simulink model "ACC_Model"  (Simulink 7.6)
settings: Solver=ode5  StartTime=0.0  StopTime=inf  FixedStep=1/100  RelTol=1e-3
undefined symbols (not defined in the file or in its folder): DiscIntNeverNeededParam
libraries: simulink x21, simulink_extras x6
(part 1 of 4)
settings Model: Creator=Krzysztof  LastModifiedBy=pastora  BufferReuse=off
settings DataIOCC: SaveOutput=off  SaveTime=off
settings OptimizationCC: InlineParams=on  OptimizeBlockIOStorage=off  BufferReuse=off  ExpressionFolding=off  LocalBlockOutputs=off
settings DebuggingCC: SaveWithDisabledLinksMsg=none  SaveWithParameterizedLinksMsg=none  SolverPrmCheckMsg=none  InheritedTsInSrcMsg=none  DiscreteInheritContinuousMsg=none  ParameterPrecisionLossMsg=none
settings ModelReferenceCC: ModelReferenceNumInstancesAllowed=Single
settings SFSimCC: SimParseCustomCode=off

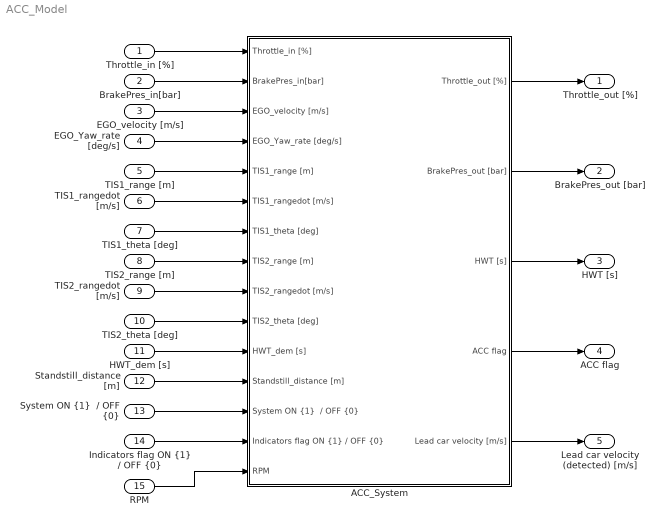
== system ACC_Model ==
  Throttle_in [%] : Inport
  BrakePres_in[bar] : Inport  Port=2
  EGO_velocity [m/s] : Inport  Port=3
  EGO_Yaw_rate [deg/s] : Inport  Port=4
  TIS1_range [m] : Inport  Port=5
  TIS1_rangedot [m/s] : Inport  Port=6
  TIS1_theta [deg] : Inport  Port=7
  TIS2_range [m] : Inport  Port=8
  TIS2_rangedot [m/s] : Inport  Port=9
  TIS2_theta [deg] : Inport  Port=10
  HWT_dem [s] : Inport  Port=11
  Standstill_distance [m] : Inport  Port=12
  "System ON {1}  / OFF {0}" : Inport  Port=13
  "Indicators flag ON {1} / OFF {0}" : Inport  Port=14
  RPM : Inport  Port=15
  ACC_System : Subsystem  mask(ACC System){J_xx=210, Rw=0.34, LaneWidth=3.5, Qfac=40.4695, BrakePressureMax=150, BrakeMax=3.5, MaxSpeed=200, drd=3, LowSpeedActv=40, TISMaxRange=[150 30], TISMaxTheta=[9 80], Tblock=1/100, TISsensor=[1/25 1/25], TISdet=[32 32], DisplaySwitch=on, DisplayFreq=25, RadarSwitch=on, RadarFreq=25}
      mask prompts: J_xx "Principal moment of inertia along longitudal (x) axis Jxx [kg*m^2]"; Rw "Tyre radius Rw [m]"; LaneWidth "Width of the lane [m]"; Qfac "Conversion factor of braking pressure into braking torque Qfac [Nm/bar]"; BrakePressureMax "Maximum brake pressure (that the controller can apply) [bar]"; BrakeMax "Maximum acceleration / deceleration, which can be applied by ACC [m/s^2]"; MaxSpeed "Maximum ACC operating velocity [km/h]"; drd "Cut-Off relatve velocity of EGO and LEAD [km/h]"; LowSpeedActv "LEAD Cut-Off Speed [km/h]"; TISMaxRange "TIS maximum range (TIS1 and TIS2) [m]"; TISMaxTheta "TIS maximum theta angle (TIS1 and TIS2) [deg]"; Tblock "Target update rate of the compilation sheet [s]"; TISsensor "TIS update rate (TIS1 and TIS2) [s]"; TISdet "TIS max. objects to detect (TIS1 and TIS2)"; DisplaySwitch "Show EGO parameters visualization"; DisplayFreq "EGO parameters visualization frequency [Hz]"; RadarSwitch "Show radar visualization"; RadarFreq "Radar frequency [Hz]"
      mask help: PreScan Experiment and Simple Dynamics model parameters
      mask init:
      | Tsensor = max([TISsensor]);
      mask CallbackString:
      | ||||||||||||||en = get_param(gcb,'MaskEnables');
      | switch get_param(gcb, 'DisplaySwitch')
      |     case 'off'
      |         en{16} = 'off';
      |     case 'on'
      |         en{16} = 'on';
      | end
      | set_param(gcb,'MaskEnables',en);||en = get_param(gcb,'MaskEnables');
      | switch get_param(gcb, 'RadarSwitch')
      |     case 'off'
      |         en{18} = 'off';
      |     case 'on'
      |         en{18} = 'on';
      | end
      | set_param(gcb,'MaskEnables',en);|
  Throttle_out [%] : Outport
  BrakePres_out [bar] : Outport  Port=2
  HWT [s] : Outport  Port=3
  ACC flag : Outport  Port=4
  Lead car velocity (detected) [m/s] : Outport  Port=5
  wires:
  "Indicators flag ON {1} / OFF {0}"/1 -> ACC_System/14("Indicators flag ON {1} / OFF {0}")
  ACC_System/1(Throttle_out [%]) -> Throttle_out [%]/1
  ACC_System/2(BrakePres_out [bar]) -> BrakePres_out [bar]/1
  ACC_System/3(HWT [s]) -> HWT [s]/1
  ACC_System/4(ACC flag) -> ACC flag/1
  ACC_System/5(Lead car velocity [m/s]) -> Lead car velocity (detected) [m/s]/1
  EGO_Yaw_rate [deg/s]/1 -> ACC_System/4(EGO_Yaw_rate [deg/s])
  TIS1_range [m]/1 -> ACC_System/5(TIS1_range [m])
  TIS1_rangedot [m/s]/1 -> ACC_System/6(TIS1_rangedot [m/s])
  TIS1_theta [deg]/1 -> ACC_System/7(TIS1_theta [deg])
  TIS2_range [m]/1 -> ACC_System/8(TIS2_range [m])
  TIS2_rangedot [m/s]/1 -> ACC_System/9(TIS2_rangedot [m/s])
  TIS2_theta [deg]/1 -> ACC_System/10(TIS2_theta [deg])
  EGO_velocity [m/s]/1 -> ACC_System/3(EGO_velocity [m/s])
  HWT_dem [s]/1 -> ACC_System/11(HWT_dem [s])
  Standstill_distance [m]/1 -> ACC_System/12(Standstill_distance [m])
  "System ON {1}  / OFF {0}"/1 -> ACC_System/13("System ON {1}  / OFF {0}")
  Throttle_in [%]/1 -> ACC_System/1(Throttle_in [%])
  BrakePres_in[bar]/1 -> ACC_System/2(BrakePres_in[bar])
  RPM/1 -> ACC_System/15(RPM)

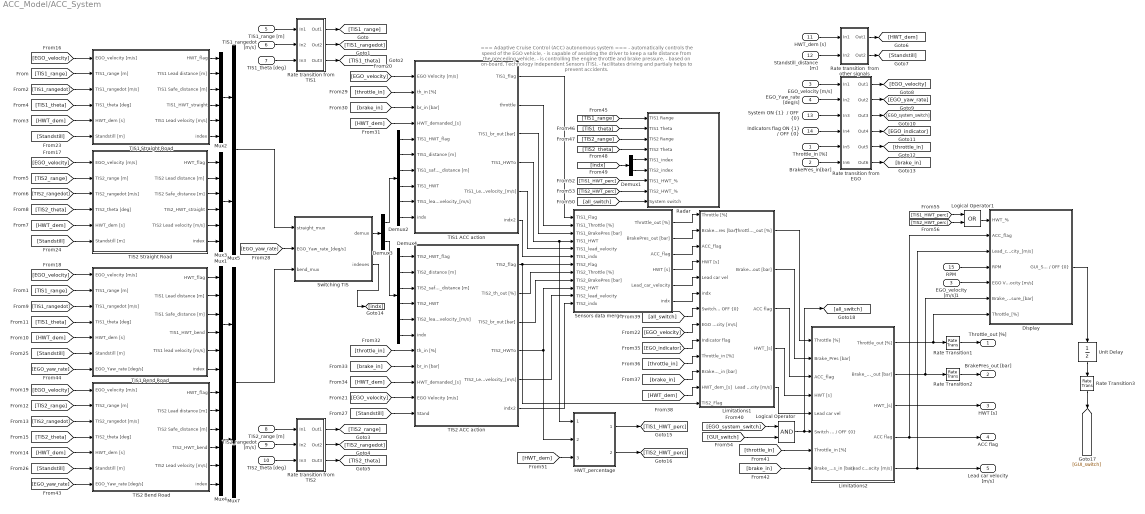
== system ACC_Model/ACC_System ==
  note: === Adaptive Cruise Control (ACC) autonomous system ===
      |
      |  - automatically controls the speed of the EGO vehicle,
      |  - is capable of assisting the driver to keep a safe distance
      |    from the preceding vehicle,
      |  - is controlling the engine throttle and brake pressure,
      |  - based on on-board, Technology Independent Sensors (TIS),
      |  - facilitates driving and partialy helps to prevent accidents.
  Throttle_in [%] : Inport  SampleTime=0
  BrakePres_in[bar] : Inport  Port=2  SampleTime=0
  EGO_velocity [m/s] : Inport  Port=3  SampleTime=Tblock
  EGO_Yaw_rate [deg/s] : Inport  Port=4  SampleTime=Tblock
  TIS1_range [m] : Inport  Port=5  PortDimensions=TISdet(1)  SampleTime=TISsensor(1)
  TIS1_rangedot [m/s] : Inport  Port=6  PortDimensions=TISdet(1)  SampleTime=TISsensor(1)
  TIS1_theta [deg] : Inport  Port=7  PortDimensions=TISdet(1)  SampleTime=TISsensor(1)
  TIS2_range [m] : Inport  Port=8  PortDimensions=TISdet(2)  SampleTime=TISsensor(2)
  TIS2_rangedot [m/s] : Inport  Port=9  PortDimensions=TISdet(2)  SampleTime=TISsensor(2)
  TIS2_theta [deg] : Inport  Port=10  PortDimensions=TISdet(2)  SampleTime=TISsensor(2)
  HWT_dem [s] : Inport  Port=11
  Standstill_distance [m] : Inport  Port=12
  "System ON {1}  / OFF {0}" : Inport  Port=13
  "Indicators flag ON {1} / OFF {0}" : Inport  Port=14
  RPM : Inport  Port=15  SampleTime=0
  Demux1 : Demux  Outputs=2
  Demux2 : Demux  Outputs=6
  Demux3 : Demux  Outputs=2
  Demux4 : Demux  Outputs=6
  Display : Subsystem
  EGO_velocity [m/s]1 : InportShadow  Port=3  SampleTime=Tblock
  HWT_percentage : Subsystem
  Limitations1 : Subsystem
  Limitations2 : Subsystem
  Logical Operator : Logic  AllPortsSameDT=off  OutDataTypeStr=boolean
  Logical Operator1 : Logic  Operator=OR  AllPortsSameDT=off  OutDataTypeStr=boolean
  Mux{1..4} (4 alike) : Mux  Inputs=6
  Mux5 : Mux  Inputs=2
  Mux7 : Mux  Inputs=2
  Radar : Subsystem
  Rate Transition1 : RateTransition  Integrity=off  OutPortSampleTime=0
  Rate Transition2 : RateTransition  Integrity=off  OutPortSampleTime=0
  Rate Transition3 : RateTransition  Integrity=off  OutPortSampleTime=Tsensor
  Rate transition  from other signals : Subsystem
  Rate transition from EGO : Subsystem
  Rate transition from TIS1 : Subsystem
  Rate transition from TIS2 : Subsystem
  Sensors data merge : Subsystem
  Switching TIS : Subsystem
  TIS1 ACC action : Subsystem
  TIS1 Bend Road : Subsystem
  TIS1 Straight Road : Subsystem
  TIS2 ACC action : Subsystem
  TIS2 Bend Road : Subsystem
  TIS2 Straight Road : Subsystem
  Unit Delay : UnitDelay  X0=1  SampleTime=-1
  Throttle_out [%] : Outport
  BrakePres_out [bar] : Outport  Port=2
  HWT [s] : Outport  Port=3
  ACC flag : Outport  Port=4
  Lead car velocity [m/s] : Outport  Port=5
  wires:
  Sensors data merge/1(Throttle_out [%]) -> Limitations1/1(Throttle [%])
  Sensors data merge/2(BrakePres_out [bar]) -> Limitations1/2(Brake_Pres [bar])
  TIS1 ACC action/1(TIS1_flag) -> Sensors data merge/1(TIS1_Flag)
  TIS1 ACC action/2(throttle) -> Sensors data merge/2(TIS1_Throttle [%])
  TIS1 ACC action/3(TIS1_br_out [bar]) -> Sensors data merge/3(TIS1_BrakePres [bar])
  TIS1 ACC action/4(TIS1_HWTo) -> Sensors data merge/4(TIS1_HWT), HWT_percentage/1(TIS1_HWT)
  Sensors data merge/3(ACC_flag) -> Limitations1/3(ACC_flag)
  Sensors data merge/4(HWT [s]) -> Limitations1/4(HWT [s])
  Sensors data merge/5(Lead_car_velocity) -> Limitations1/5(Lead car vel)
  TIS1 ACC action/5(TIS1_Lead_velocity_[m/s]) -> Sensors data merge/5(TIS1_lead_velocity)
  TIS2 ACC action/1(TIS2_flag) -> Sensors data merge/7(TIS2_Flag), Limitations1/13(TIS2_Flag)
  TIS2 ACC action/2(TIS2_th_out [%]) -> Sensors data merge/8(TIS2_Throttle [%])
  TIS2 ACC action/3(TIS2_br_out [bar]) -> Sensors data merge/9(TIS2_BrakePres [bar])
  TIS2 ACC action/4(TIS2_HWTo) -> Sensors data merge/10(TIS2_HWT), HWT_percentage/2(TIS2_HWT)
  TIS2 ACC action/5(TIS2_Lead_velocity_[m/s]) -> Sensors data merge/11(TIS2_lead_velocity)
  TIS1 Straight Road/1(HWT_flag) -> Mux2/1
  TIS1 Straight Road/2(TIS1 Lead distance [m]) -> Mux2/2
  TIS1 Straight Road/3(TIS1 Safe_distance [m]) -> Mux2/3
  TIS1 Straight Road/4(TIS1_HWT_straight) -> Mux2/4
  TIS1 Straight Road/5(TIS1 Lead velocity [m/s]) -> Mux2/5
  TIS1 Straight Road/6(index) -> Mux2/6
  TIS1 ACC action/6(indx2) -> Sensors data merge/6(TIS1_indx)
  TIS2 ACC action/6(indx2) -> Sensors data merge/12(TIS2_indx)
  Sensors data merge/6(indx) -> Limitations1/6(indx)
  Limitations1/1(Throttle_out [%]) -> Limitations2/1(Throttle [%])
  Limitations1/2(Brake_Pres_out [bar]) -> Limitations2/2(Brake_Pres [bar])
  Limitations1/4(HWT_[s]) -> Limitations2/4(HWT [s])
  Limitations1/3(ACC flag) -> Limitations2/3(ACC_flag)
  Limitations1/5(Lead car velocity [m/s]) -> Limitations2/5(Lead car vel)
  TIS1_range [m]/1 -> Rate transition from TIS1/1(In1)
  TIS1_rangedot [m/s]/1 -> Rate transition from TIS1/2(In2)
  TIS1_theta [deg]/1 -> Rate transition from TIS1/3(In3)
  TIS2_range [m]/1 -> Rate transition from TIS2/1(In1)
  TIS2_rangedot [m/s]/1 -> Rate transition from TIS2/2(In2)
  TIS2_theta [deg]/1 -> Rate transition from TIS2/3(In3)
  Rate transition from TIS1/1(Out1) -> [TIS1_range]
  Rate transition from TIS1/2(Out2) -> [TIS1_rangedot]
  Rate transition from TIS1/3(Out3) -> [TIS1_theta]
  Rate transition from TIS2/1(Out1) -> [TIS2_range]
  Rate transition from TIS2/2(Out2) -> [TIS2_rangedot]
  Rate transition from TIS2/3(Out3) -> [TIS2_theta]
  [TIS1_range] -> TIS1 Straight Road/2(TIS1_range [m])
  [TIS1_rangedot] -> TIS1 Straight Road/3(TIS1_rangedot [m/s])
  [TIS1_theta] -> TIS1 Straight Road/4(TIS1_theta [deg])
  [TIS2_range] -> TIS2 Straight Road/2(TIS2_range [m])
  [TIS2_rangedot] -> TIS2 Straight Road/3(TIS2_rangedot [m/s])
  [TIS2_theta] -> TIS2 Straight Road/4(TIS2_theta [deg])
  [TIS1_range] -> TIS1 Bend Road/2(TIS1_range [m])
  [TIS1_rangedot] -> TIS1 Bend Road/3(TIS1_rangedot [m/s])
  [TIS1_theta] -> TIS1 Bend Road/4(TIS1_theta [deg])
  [TIS2_range] -> TIS2 Bend Road/2(TIS2_range [m])
  [TIS2_rangedot] -> TIS2 Bend Road/3(TIS2_rangedot [m/s])
  [TIS2_theta] -> TIS2 Bend Road/4(TIS2_theta [deg])
  EGO_velocity [m/s]/1 -> Rate transition from EGO/1(In1)
  EGO_Yaw_rate [deg/s]/1 -> Rate transition from EGO/2(In2)
  HWT_dem [s]/1 -> Rate transition  from other signals/1(In1)
  Standstill_distance [m]/1 -> Rate transition  from other signals/2(In2)
  "System ON {1}  / OFF {0}"/1 -> Rate transition from EGO/3(In3)
  Throttle_in [%]/1 -> Rate transition from EGO/5(In5)
  BrakePres_in[bar]/1 -> Rate transition from EGO/6(In6)
  "Indicators flag ON {1} / OFF {0}"/1 -> Rate transition from EGO/4(In4)
  Rate transition  from other signals/1(Out1) -> [HWT_dem]
  Rate transition  from other signals/2(Out2) -> [Standstill]
  [HWT_dem] -> TIS1 Straight Road/5(HWT_dem [s])
  [HWT_dem] -> TIS2 Straight Road/5(HWT_dem [s])
  [HWT_dem] -> TIS1 Bend Road/5(HWT_dem [s])
  [HWT_dem] -> TIS2 Bend Road/5(HWT_dem [s])
  Rate transition from EGO/1(Out1) -> [EGO_velocity]
  Rate transition from EGO/2(Out2) -> [EGO_yaw_rate]
  Rate transition from EGO/3(Out3) -> [EGO_system_switch]
  Rate transition from EGO/4(Out4) -> [EGO_indicator]
  Rate transition from EGO/5(Out5) -> [throttle_in]
  Rate transition from EGO/6(Out6) -> [brake_in]
  [EGO_velocity] -> TIS1 Straight Road/1(EGO_velocity [m/s])
  [EGO_velocity] -> TIS2 Straight Road/1(EGO_velocity [m/s])
  [EGO_velocity] -> TIS1 Bend Road/1(EGO_velocity [m/s])
  [EGO_velocity] -> TIS2 Bend Road/1(EGO_velocity [m/s])
  [EGO_velocity] -> TIS1 ACC action/1(EGO Velocity [m/s])
  [EGO_velocity] -> TIS2 ACC action/10(EGO Velocity [m/s])
  [EGO_velocity] -> Limitations1/8(EGO Velocity [m/s])
  [Standstill] -> TIS1 Straight Road/6(Standstill [m])
  [Standstill] -> TIS2 Straight Road/6(Standstill [m])
  [Standstill] -> TIS1 Bend Road/6(Standstill [m])
  [Standstill] -> TIS2 Bend Road/6(Standstill [m])
  [Standstill] -> TIS2 ACC action/11(Stand)
  [EGO_yaw_rate] -> Switching TIS/2(EGO_Yaw_rate_[deg/s])
  [throttle_in] -> TIS1 ACC action/2(th_in [%])
  [brake_in] -> TIS1 ACC action/3(br_in [bar])
  [HWT_dem] -> TIS1 ACC action/4(HWT_demanded_[s])
  [throttle_in] -> TIS2 ACC action/7(th_in [%])
  [brake_in] -> TIS2 ACC action/8(br_in [bar])
  [HWT_dem] -> TIS2 ACC action/9(HWT_demanded_[s])
  [EGO_indicator] -> Limitations1/9(Indicator flag)
  [throttle_in] -> Limitations1/10(Throttle_in [%])
  [brake_in] -> Limitations1/11(Brake_Pres_in [bar])
  [HWT_dem] -> Limitations1/12(HWT_dem_[s])
  [all_switch] -> Limitations1/7("Switch ON {1} / OFF {0}")
  [throttle_in] -> Limitations2/7(Throttle_in [%])
  [brake_in] -> Limitations2/8(Brake_Pres_in [bar])
  [EGO_yaw_rate] -> TIS2 Bend Road/7(EGO_Yaw_rate [deg/s])
  [EGO_yaw_rate] -> TIS1 Bend Road/7(EGO_Yaw_rate [deg/s])
  Limitations2/1(Throttle_out [%]) -> Rate Transition1/1, Display/7(Throttle_[%])
  Limitations2/2(Brake_Pres_out [bar]) -> Rate Transition2/1, Display/6(Brake_Pressure_[bar])
  Rate Transition1/1 -> Throttle_out [%]/1
  Rate Transition2/1 -> BrakePres_out [bar]/1
  Limitations2/3(HWT_[s]) -> HWT [s]/1
  Limitations2/4(ACC flag) -> ACC flag/1, Display/2(ACC_flag)
  Limitations2/5(Lead car velocity [m/s]) -> Lead car velocity [m/s]/1, Display/3(Lead_car_velocity_[m/s])
  [TIS1_range] -> Radar/1(TIS1 Range)
  [TIS1_theta] -> Radar/2(TIS1 Theta)
  [TIS2_range] -> Radar/3(TIS2 Range)
  [TIS2_theta] -> Radar/4(TIS2 Theta)
  Mux2/1 -> Mux5/1
  TIS2 Straight Road/1(HWT_flag) -> Mux3/1
  TIS2 Straight Road/2(TIS2 Lead distance [m]) -> Mux3/2
  TIS2 Straight Road/3(TIS2 Safe_distance [m]) -> Mux3/3
  TIS2 Straight Road/4(TIS2_HWT_straight) -> Mux3/4
  TIS2 Straight Road/5(TIS2 Lead velocity [m/s]) -> Mux3/5
  TIS2 Straight Road/6(index) -> Mux3/6
  Mux3/1 -> Mux5/2
  TIS2 Bend Road/1(HWT_flag) -> Mux4/1
  TIS2 Bend Road/2(TIS2 Lead distance [m]) -> Mux4/2
  TIS2 Bend Road/3(TIS2 Safe_distance [m]) -> Mux4/3
  TIS2 Bend Road/4(TIS2_HWT_bend) -> Mux4/4
  TIS2 Bend Road/5(TIS2 Lead velocity [m/s]) -> Mux4/5
  TIS2 Bend Road/6(index) -> Mux4/6
  Mux5/1 -> Switching TIS/1(straight_mux)
  TIS1 Bend Road/1(HWT_flag) -> Mux1/1
  TIS1 Bend Road/2(TIS1 Lead distance [m]) -> Mux1/2
  TIS1 Bend Road/3(TIS1 Safe_distance [m]) -> Mux1/3
  TIS1 Bend Road/4(TIS1_HWT_bend) -> Mux1/4
  TIS1 Bend Road/5(TIS1 lead velocity [m/s]) -> Mux1/5
  TIS1 Bend Road/6(index) -> Mux1/6
  Mux1/1 -> Mux7/1
  Mux4/1 -> Mux7/2
  Mux7/1 -> Switching TIS/3(bend_mux)
  Switching TIS/2(indexes) -> [indx]
  Demux1/1 -> Radar/5(TIS1_index)
  Demux1/2 -> Radar/6(TIS2_index)
  [indx] -> Demux1/1
  Switching TIS/1(demux) -> Demux3/1
  Demux2/1 -> TIS1 ACC action/5(TIS1_HWT_flag)
  Demux2/2 -> TIS1 ACC action/6(TIS1_distance [m])
  Demux2/3 -> TIS1 ACC action/7(TIS1_safe_distance [m])
  Demux2/4 -> TIS1 ACC action/8(TIS1_HWT)
  Demux2/5 -> TIS1 ACC action/9(TIS1_lead_velocity_[m/s])
  Demux2/6 -> TIS1 ACC action/10(indx)
  Demux3/1 -> Demux2/1
  Demux4/1 -> TIS2 ACC action/1(TIS2_HWT_flag)
  Demux4/2 -> TIS2 ACC action/2(TIS2_distance [m])
  Demux4/3 -> TIS2 ACC action/3(TIS2_safe_distance [m])
  Demux4/4 -> TIS2 ACC action/4(TIS2_HWT)
  Demux4/5 -> TIS2 ACC action/5(TIS2_lead_velocity_[m/s])
  Demux4/6 -> TIS2 ACC action/6(indx)
  Demux3/2 -> Demux4/1
  [HWT_dem] -> HWT_percentage/3(HWT_dem_[s])
  HWT_percentage/1(TIS1_HWT_perc) -> [TIS1_HWT_perc]
  HWT_percentage/2(TIS2_HWT_perc) -> [TIS2_HWT_perc]
  [TIS1_HWT_perc] -> Radar/7(TIS1_HWT_%)
  [TIS2_HWT_perc] -> Radar/8(TIS2_HWT_%)
  Display/1("GUI_System ON {1} / OFF {0}") -> Unit Delay/1
  RPM/1 -> Display/4(RPM)
  EGO_velocity [m/s]1/1 -> Display/5(EGO Velocity [m/s])
  Unit Delay/1 -> Rate Transition3/1
  Rate Transition3/1 -> [GUI_switch]
  Logical Operator/1 -> Limitations2/6("Switch ON {1} / OFF {0}"), [all_switch]
  [EGO_system_switch] -> Logical Operator/1
  [GUI_switch] -> Logical Operator/2
  [all_switch] -> Radar/9(System switch)
  [TIS1_HWT_perc] -> Logical Operator1/1
  [TIS2_HWT_perc] -> Logical Operator1/2
  Logical Operator1/1 -> Display/1(HWT_%)

== system ACC_Model/ACC_System/Display ==
  HWT_% : Inport
  ACC_flag : Inport  Port=2
  Lead_car_velocity_[m/s] : Inport  Port=3
  RPM : Inport  Port=4
  EGO Velocity [m/s] : Inport  Port=5
  Brake_Pressure_[bar] : Inport  Port=6
  Throttle_[%] : Inport  Port=7
  Display switch : Constant  Value=DisplaySwitch
  If : If
  If Action Subsystem : Subsystem  TreatAsAtomicUnit=on
  If Action Subsystem1 : Subsystem  TreatAsAtomicUnit=on
  Merge : Merge  InitialOutput=1
  Rate Transition : RateTransition  Integrity=off  OutPortSampleTime=Tsensor
  Rate Transition{1..6,8} (7 alike) : RateTransition  Integrity=off  OutPortSampleTime=1/DisplayFreq
  "GUI_System ON {1} / OFF {0}" : Outport
  wires:
  RPM/1 -> Rate Transition1/1
  EGO Velocity [m/s]/1 -> Rate Transition2/1
  Brake_Pressure_[bar]/1 -> Rate Transition3/1
  HWT_%/1 -> Rate Transition4/1
  ACC_flag/1 -> Rate Transition5/1
  Lead_car_velocity_[m/s]/1 -> Rate Transition6/1
  Throttle_[%]/1 -> Rate Transition8/1
  Display switch/1 -> If/1
  Rate Transition1/1 -> If Action Subsystem/1(RPM1)
  Rate Transition2/1 -> If Action Subsystem/2(EGO Velocity [m/s]1)
  Rate Transition3/1 -> If Action Subsystem/3(Brake_Pressure_[bar]1)
  Rate Transition4/1 -> If Action Subsystem/4(HWT_%1)
  Rate Transition5/1 -> If Action Subsystem/5(ACC_flag1)
  Rate Transition6/1 -> If Action Subsystem/6(Lead_car_velocity_[m/s]1)
  Rate Transition8/1 -> If Action Subsystem/7(Throttle_[%]1)
  If/1 -> If Action Subsystem/Action
  If Action Subsystem/1("GUI_System ON {1} / OFF {0}1") -> Merge/1
  If Action Subsystem1/1(Out1) -> Merge/2
  If/2 -> If Action Subsystem1/Action
  Merge/1 -> Rate Transition/1
  Rate Transition/1 -> "GUI_System ON {1} / OFF {0}"/1

== system ACC_Model/ACC_System/HWT_percentage ==
  TIS1_HWT : Inport
  TIS2_HWT : Inport  Port=2  SampleTime=Tsensor
  HWT_dem_[s] : Inport  Port=3  SampleTime=Tsensor
  Bias : Bias  Bias=-1
  Brake Pressure [ar]1 : Gain  Gain=100
  Constant : Constant  Value=10
  Constant1 : Constant  Value=0
  Demux : Demux  Outputs=2
  Divide : Product  Inputs=*/
  Logical Operator : Logic  AllPortsSameDT=off  OutDataTypeStr=boolean
  Mux : Mux  Inputs=2
  Relational Operator : RelationalOperator  Operator=<  OutDataTypeStr=boolean
  Relational Operator1 : RelationalOperator  Operator=>  OutDataTypeStr=boolean
  TIS1_HWT_perc : Outport
  TIS2_HWT_perc : Outport  Port=2
  wires:
  Divide/1 -> Bias/1
  Bias/1 -> Brake Pressure [ar]1/1
  TIS1_HWT/1 -> Mux/1
  TIS2_HWT/1 -> Mux/2
  Brake Pressure [ar]1/1 -> Relational Operator/1
  Constant/1 -> Relational Operator/2
  Mux/1 -> Divide/1, Relational Operator1/1
  HWT_dem_[s]/1 -> Divide/2
  Demux/1 -> TIS1_HWT_perc/1
  Demux/2 -> TIS2_HWT_perc/1
  Relational Operator/1 -> Logical Operator/1
  Logical Operator/1 -> Demux/1
  Relational Operator1/1 -> Logical Operator/2
  Constant1/1 -> Relational Operator1/2

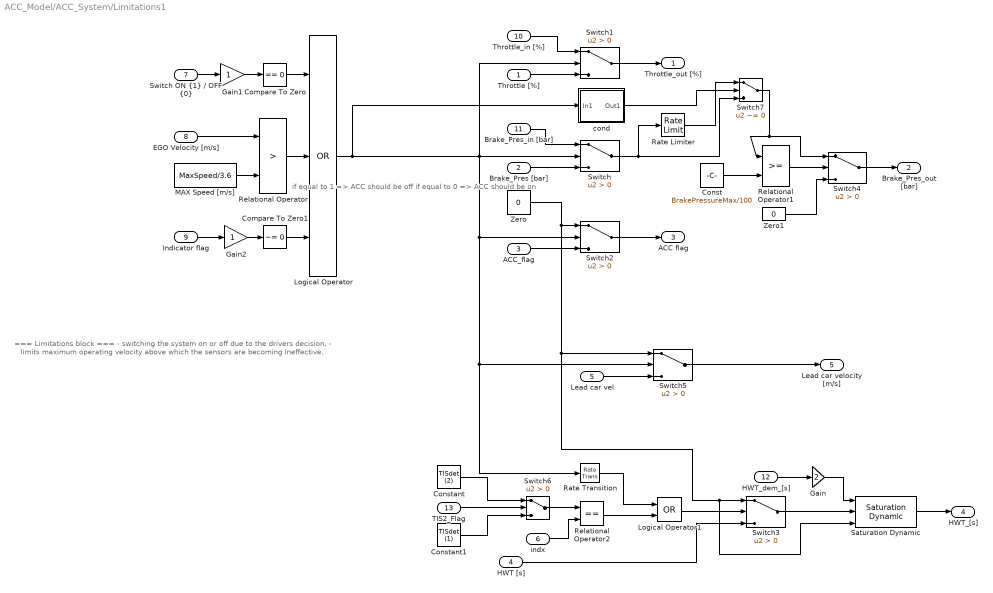
== system ACC_Model/ACC_System/Limitations1 ==
  note: if equal to 1 => ACC should be off
      | if equal to 0 => ACC should be on
  note: === Limitations block ===
      |
      |  - switching the system on or off due to the drivers decision,
      |  - limits maximum operating velocity
      |    above which the sensors are becoming ineffective.
  Throttle [%] : Inport
  Brake_Pres [bar] : Inport  Port=2
  ACC_flag : Inport  Port=3
  HWT [s] : Inport  Port=4
  Lead car vel : Inport  Port=5
  indx : Inport  Port=6
  "Switch ON {1} / OFF {0}" : Inport  Port=7
  EGO Velocity [m/s] : Inport  Port=8
  Indicator flag : Inport  Port=9
  Throttle_in [%] : Inport  Port=10
  Brake_Pres_in [bar] : Inport  Port=11
  HWT_dem_[s] : Inport  Port=12
  TIS2_Flag : Inport  Port=13
  Compare To Zero : simulink/Logic and Bit Operations/Compare To Zero  SystemSampleTime=-1  relop===  LogicOutDataTypeMode=boolean
  Compare To Zero1 : simulink/Logic and Bit Operations/Compare To Zero  SystemSampleTime=-1  relop=~=  LogicOutDataTypeMode=boolean
  Const : Constant  Value=BrakePressureMax/100
  Constant : Constant  Value=TISdet (2)
  Constant1 : Constant  Value=TISdet (1)
  Gain : Gain  Gain=2
  Gain1 : Gain
  Gain2 : Gain
  Logical Operator : Logic  Operator=OR  Inputs=3  AllPortsSameDT=off  OutDataTypeStr=boolean
  Logical Operator1 : Logic  Operator=OR  AllPortsSameDT=off  OutDataTypeStr=boolean
  MAX Speed [m/s] : Constant  Value=MaxSpeed/3.6
  Rate Limiter : RateLimiter  RisingSlewLimit=BrakePressureMax  FallingSlewLimit=-BrakePressureMax  SampleTimeMode=inherited
  Rate Transition : RateTransition  Integrity=off  OutPortSampleTime=Tsensor
  Relational Operator : RelationalOperator  Operator=>  OutDataTypeStr=boolean
  Relational Operator1 : RelationalOperator  OutDataTypeStr=boolean
  Relational Operator2 : RelationalOperator  Operator===  OutDataTypeStr=boolean
  Saturation Dynamic : simulink/Discontinuities/Saturation Dynamic  SystemSampleTime=-1  OutMin=[]  OutMax=[]  OutDataTypeStr=Inherit: Same as second input  OutDataType=fixdt(1, 16)  OutScaling=2^-10  DoSatur=off
  Switch{,1..6} (7 alike) : Switch  Criteria=u2 > Threshold
  Switch7 : Switch  Criteria=u2 ~= 0
  Zero : Constant  Value=0
  Zero1 : Constant  Value=0
  cond : Subsystem
  Throttle_out [%] : Outport
  Brake_Pres_out [bar] : Outport  Port=2
  ACC flag : Outport  Port=3
  HWT_[s] : Outport  Port=4
  Lead car velocity [m/s] : Outport  Port=5
  wires:
  EGO Velocity [m/s]/1 -> Relational Operator/1
  MAX Speed [m/s]/1 -> Relational Operator/2
  "Switch ON {1} / OFF {0}"/1 -> Gain1/1
  Indicator flag/1 -> Gain2/1
  Logical Operator/1 -> cond/1(In1), Switch1/2, Switch2/2, Switch5/2, Rate Transition/1, Switch/2
  Throttle_in [%]/1 -> Switch1/1
  Zero/1 -> Switch2/1, Switch5/1, Switch3/1, Saturation Dynamic/3
  Throttle [%]/1 -> Switch1/3
  ACC_flag/1 -> Switch2/3
  Switch1/1 -> Throttle_out [%]/1
  Switch2/1 -> ACC flag/1
  Compare To Zero/1 -> Logical Operator/1
  Relational Operator/1 -> Logical Operator/2
  Compare To Zero1/1 -> Logical Operator/3
  HWT_dem_[s]/1 -> Gain/1
  Gain/1 -> Saturation Dynamic/1
  Gain1/1 -> Compare To Zero/1
  Gain2/1 -> Compare To Zero1/1
  Switch5/1 -> Lead car velocity [m/s]/1
  Lead car vel/1 -> Switch5/3
  indx/1 -> Relational Operator2/2
  Logical Operator1/1 -> Switch3/2
  HWT [s]/1 -> Switch3/3
  Switch3/1 -> Saturation Dynamic/2
  Saturation Dynamic/1 -> HWT_[s]/1
  Const/1 -> Relational Operator1/2
  Relational Operator1/1 -> Switch4/2
  Zero1/1 -> Switch4/3
  Switch4/1 -> Brake_Pres_out [bar]/1
  Rate Transition/1 -> Logical Operator1/1
  TIS2_Flag/1 -> Switch6/2
  Switch6/1 -> Relational Operator2/1
  Constant/1 -> Switch6/1
  Constant1/1 -> Switch6/3
  Relational Operator2/1 -> Logical Operator1/2
  Brake_Pres_in [bar]/1 -> Switch/1
  Brake_Pres [bar]/1 -> Switch/3
  cond/1(Out1) -> Switch7/2
  Switch7/1 -> Relational Operator1/1, Switch4/1
  Switch/1 -> Switch7/3, Rate Limiter/1
  Rate Limiter/1 -> Switch7/1

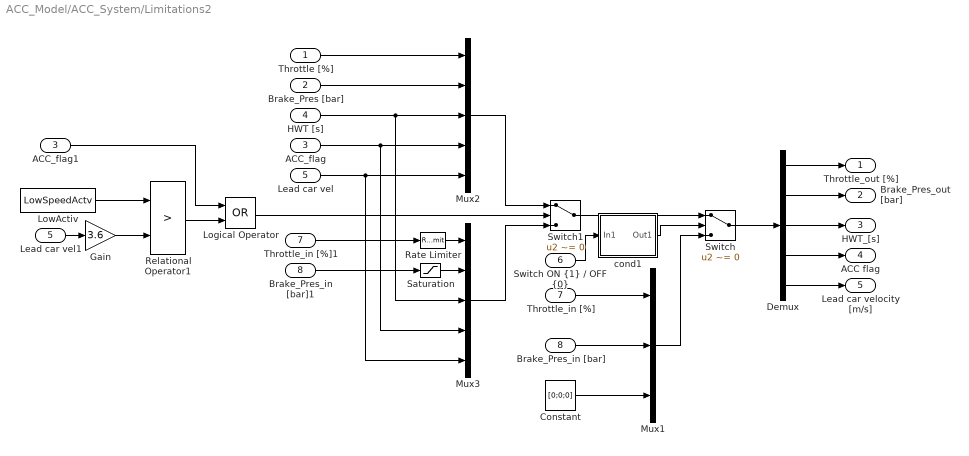
== system ACC_Model/ACC_System/Limitations2 ==
  Throttle [%] : Inport
  Brake_Pres [bar] : Inport  Port=2
  ACC_flag : Inport  Port=3
  HWT [s] : Inport  Port=4
  Lead car vel : Inport  Port=5
  "Switch ON {1} / OFF {0}" : Inport  Port=6
  Throttle_in [%] : Inport  Port=7
  Brake_Pres_in [bar] : Inport  Port=8
  ACC_flag1 : InportShadow  Port=3
  Brake_Pres_in [bar]1 : InportShadow  Port=8
  Constant : Constant  Value=[0;0;0]
  Demux : Demux  Outputs=5
  Gain : Gain  Gain=3.6
  Lead car vel1 : InportShadow  Port=5
  Logical Operator : Logic  Operator=OR  AllPortsSameDT=off  OutDataTypeStr=boolean
  LowActiv : Constant  Value=LowSpeedActv
  Mux1 : Mux  Inputs=3
  Mux2 : Mux  Inputs=5
  Mux3 : Mux  Inputs=5
  Rate Limiter : RateLimiter  RisingSlewLimit=BrakeMax*1e3  FallingSlewLimit=-BrakeMax*1e3  SampleTimeMode=inherited
  Relational Operator1 : RelationalOperator  Operator=>  OutDataTypeStr=boolean
  Saturation : Saturate  UpperLimit=BrakePressureMax  LowerLimit=0
  Switch : Switch  Criteria=u2 ~= 0
  Switch1 : Switch  Criteria=u2 ~= 0
  Throttle_in [%]1 : InportShadow  Port=7
  cond1 : Subsystem
  Throttle_out [%] : Outport
  Brake_Pres_out [bar] : Outport  Port=2
  HWT_[s] : Outport  Port=3
  ACC flag : Outport  Port=4
  Lead car velocity [m/s] : Outport  Port=5
  wires:
  "Switch ON {1} / OFF {0}"/1 -> cond1/1(In1)
  Throttle_in [%]/1 -> Mux1/1
  Brake_Pres_in [bar]/1 -> Mux1/2
  Constant/1 -> Mux1/3
  Mux1/1 -> Switch/3
  Throttle [%]/1 -> Mux2/1
  Brake_Pres [bar]/1 -> Mux2/2
  HWT [s]/1 -> Mux2/3, Mux3/3
  ACC_flag/1 -> Mux2/4, Mux3/4
  Lead car vel/1 -> Mux2/5, Mux3/5
  Mux2/1 -> Switch1/1
  Rate Limiter/1 -> Mux3/1
  Saturation/1 -> Mux3/2
  Mux3/1 -> Switch1/3
  Switch1/1 -> Switch/1
  Switch/1 -> Demux/1
  Demux/1 -> Throttle_out [%]/1
  Demux/2 -> Brake_Pres_out [bar]/1
  Demux/3 -> HWT_[s]/1
  Demux/4 -> ACC flag/1
  Demux/5 -> Lead car velocity [m/s]/1
  Throttle_in [%]1/1 -> Rate Limiter/1
  Brake_Pres_in [bar]1/1 -> Saturation/1
  LowActiv/1 -> Relational Operator1/1
  Gain/1 -> Relational Operator1/2
  Lead car vel1/1 -> Gain/1
  Logical Operator/1 -> Switch1/2
  ACC_flag1/1 -> Logical Operator/1
  Relational Operator1/1 -> Logical Operator/2
  cond1/1(Out1) -> Switch/2

== system ACC_Model/ACC_System/Radar ==
  TIS1 Range : Inport
  TIS1 Theta : Inport  Port=2
  TIS2 Range : Inport  Port=3
  TIS2 Theta : Inport  Port=4
  TIS1_index : Inport  Port=5
  TIS2_index : Inport  Port=6
  TIS1_HWT_% : Inport  Port=7
  TIS2_HWT_% : Inport  Port=8
  System switch : Inport  Port=9
  Radar : Subsystem
  Radar switch : Constant  Value=RadarSwitch
  Rate Transition{1..6,8..10} (9 alike) : RateTransition  Integrity=off  OutPortSampleTime=1/RadarFreq
  wires:
  TIS1 Range/1 -> Rate Transition5/1
  TIS1 Theta/1 -> Rate Transition1/1
  TIS2 Range/1 -> Rate Transition2/1
  TIS2 Theta/1 -> Rate Transition3/1
  Rate Transition5/1 -> Radar/1(TIS1 Range)
  Rate Transition1/1 -> Radar/2(TIS1 Theta)
  Rate Transition2/1 -> Radar/3(TIS2 Range)
  Rate Transition3/1 -> Radar/4(TIS2 Theta)
  Radar switch/1 -> Radar/Enable
  Rate Transition8/1 -> Radar/5(TIS1_index)
  TIS1_index/1 -> Rate Transition8/1
  TIS1_HWT_%/1 -> Rate Transition9/1
  TIS2_HWT_%/1 -> Rate Transition10/1
  Rate Transition9/1 -> Radar/7(TIS1_HWT_%)
  Rate Transition10/1 -> Radar/8(TIS2_HWT_%)
  TIS2_index/1 -> Rate Transition4/1
  Rate Transition4/1 -> Radar/6(TIS2_index)
  System switch/1 -> Rate Transition6/1
  Rate Transition6/1 -> Radar/9(System switch)

== system ACC_Model/ACC_System/Rate transition  from other signals ==
  In1 : Inport
  In2 : Inport  Port=2
  Rate Transition1 : RateTransition  Integrity=off  OutPortSampleTime=Tsensor
  Rate Transition2 : RateTransition  Integrity=off  OutPortSampleTime=Tsensor
  Out1 : Outport
  Out2 : Outport  Port=2
  wires:
  Rate Transition2/1 -> Out2/1
  In2/1 -> Rate Transition2/1
  Rate Transition1/1 -> Out1/1
  In1/1 -> Rate Transition1/1

== system ACC_Model/ACC_System/Rate transition from EGO ==
  In1 : Inport
  In2 : Inport  Port=2
  In3 : Inport  Port=3
  In4 : Inport  Port=4
  In5 : Inport  Port=5
  In6 : Inport  Port=6
  Rate Transition{1..6} (6 alike) : RateTransition  Integrity=off  OutPortSampleTime=Tsensor
  Out1 : Outport
  Out2 : Outport  Port=2
  Out3 : Outport  Port=3
  Out4 : Outport  Port=4
  Out5 : Outport  Port=5
  Out6 : Outport  Port=6
  wires:
  In1/1 -> Rate Transition1/1
  Rate Transition1/1 -> Out1/1
  In2/1 -> Rate Transition2/1
  Rate Transition2/1 -> Out2/1
  In3/1 -> Rate Transition3/1
  Rate Transition3/1 -> Out3/1
  In4/1 -> Rate Transition4/1
  Rate Transition4/1 -> Out4/1
  In5/1 -> Rate Transition5/1
  Rate Transition5/1 -> Out5/1
  In6/1 -> Rate Transition6/1
  Rate Transition6/1 -> Out6/1

== system ACC_Model/ACC_System/Rate transition from TIS1 ==
  In1 : Inport
  In2 : Inport  Port=2
  In3 : Inport  Port=3
  Rate Transition1 : RateTransition  Integrity=off  OutPortSampleTime=Tsensor
  Rate Transition2 : RateTransition  Integrity=off  OutPortSampleTime=Tsensor
  Rate Transition3 : RateTransition  Integrity=off  OutPortSampleTime=Tsensor
  Out1 : Outport
  Out2 : Outport  Port=2
  Out3 : Outport  Port=3
  wires:
  Rate Transition3/1 -> Out3/1
  In3/1 -> Rate Transition3/1
  Rate Transition2/1 -> Out2/1
  In2/1 -> Rate Transition2/1
  Rate Transition1/1 -> Out1/1
  In1/1 -> Rate Transition1/1

== system ACC_Model/ACC_System/Rate transition from TIS2 ==
  In1 : Inport
  In2 : Inport  Port=2
  In3 : Inport  Port=3
  Rate Transition1 : RateTransition  Integrity=off  OutPortSampleTime=Tsensor
  Rate Transition2 : RateTransition  Integrity=off  OutPortSampleTime=Tsensor
  Rate Transition3 : RateTransition  Integrity=off  OutPortSampleTime=Tsensor
  Out1 : Outport
  Out2 : Outport  Port=2
  Out3 : Outport  Port=3
  wires:
  In1/1 -> Rate Transition3/1
  Rate Transition3/1 -> Out1/1
  In2/1 -> Rate Transition1/1
  Rate Transition1/1 -> Out2/1
  In3/1 -> Rate Transition2/1
  Rate Transition2/1 -> Out3/1

== system ACC_Model/ACC_System/Sensors data merge ==
  note: === Sensors data merge block ===
      |
      |  - merges data from both sensors,
      |  - chooses the second, short - range sensor as major,
      |  - limits acceleration and deceleration of the EGO car.
  TIS1_Flag : Inport
  TIS1_Throttle [%] : Inport  Port=2
  TIS1_BrakePres [bar] : Inport  Port=3
  TIS1_HWT : Inport  Port=4
  TIS1_lead_velocity : Inport  Port=5
  TIS1_indx : Inport  Port=6
  TIS2_Flag : Inport  Port=7
  TIS2_Throttle [%] : Inport  Port=8
  TIS2_BrakePres [bar] : Inport  Port=9
  TIS2_HWT : Inport  Port=10
  TIS2_lead_velocity : Inport  Port=11
  TIS2_indx : Inport  Port=12
  Rate Limiter : RateLimiter  RisingSlewLimit=16  FallingSlewLimit=-inf  SampleTimeMode=inherited
  Saturation : Saturate  UpperLimit=100  LowerLimit=0
  Saturation1 : Saturate  UpperLimit=BrakePressureMax  LowerLimit=0
  Switch{,1,3..6} (6 alike) : Switch  Criteria=u2 > Threshold
  Switch2 : Switch  Criteria=u2 ~= 0
  Throttle_out [%] : Outport
  BrakePres_out [bar] : Outport  Port=2
  ACC_flag : Outport  Port=3
  HWT [s] : Outport  Port=4
  Lead_car_velocity : Outport  Port=5
  indx : Outport  Port=6
  wires:
  TIS2_Flag/1 -> Switch/2, Switch1/2, Switch3/1, Switch3/2, Switch4/2, Switch6/2, Switch5/2
  TIS2_Throttle [%]/1 -> Switch/1
  TIS2_BrakePres [bar]/1 -> Switch1/1
  TIS1_Throttle [%]/1 -> Switch/3
  TIS1_BrakePres [bar]/1 -> Switch1/3
  Switch/1 -> Saturation/1
  Switch1/1 -> Saturation1/1, Switch2/2
  Switch2/1 -> Throttle_out [%]/1
  Saturation/1 -> Switch2/1, Rate Limiter/1
  Rate Limiter/1 -> Switch2/3
  TIS1_Flag/1 -> Switch3/3
  Switch3/1 -> ACC_flag/1
  Switch4/1 -> HWT [s]/1
  TIS2_HWT/1 -> Switch4/1
  TIS1_HWT/1 -> Switch4/3
  Saturation1/1 -> BrakePres_out [bar]/1
  TIS2_lead_velocity/1 -> Switch6/1
  TIS1_lead_velocity/1 -> Switch6/3
  Switch6/1 -> Lead_car_velocity/1
  TIS2_indx/1 -> Switch5/1
  TIS1_indx/1 -> Switch5/3
  Switch5/1 -> indx/1

== system ACC_Model/ACC_System/Switching TIS ==
  note: === Switching block ===
      |
      |  - determines if the EGO car is moving on a straight road or on a bend raod,
      |  - based on the actual value of the yaw rate of the EGO car.
  straight_mux : Inport
  EGO_Yaw_rate_[deg/s] : Inport  Port=2
  bend_mux : Inport  Port=3
  1deg_per_s : Constant
  Abs : Abs
  Relational Operator : RelationalOperator  Operator=<  OutDataTypeStr=boolean
  Selector : Selector  InputPortWidth=12  IndexOptions=Index vector (dialog)  Indices=[6 12]  OutputSizes=1
  Switch : Switch  Criteria=u2 ~= 0  Threshold=0.5
  demux : Outport
  indexes : Outport  Port=2
  wires:
  EGO_Yaw_rate_[deg/s]/1 -> Abs/1
  1deg_per_s/1 -> Relational Operator/2
  Relational Operator/1 -> Switch/2
  straight_mux/1 -> Switch/1
  Switch/1 -> demux/1, Selector/1
  bend_mux/1 -> Switch/3
  Abs/1 -> Relational Operator/1
  Selector/1 -> indexes/1

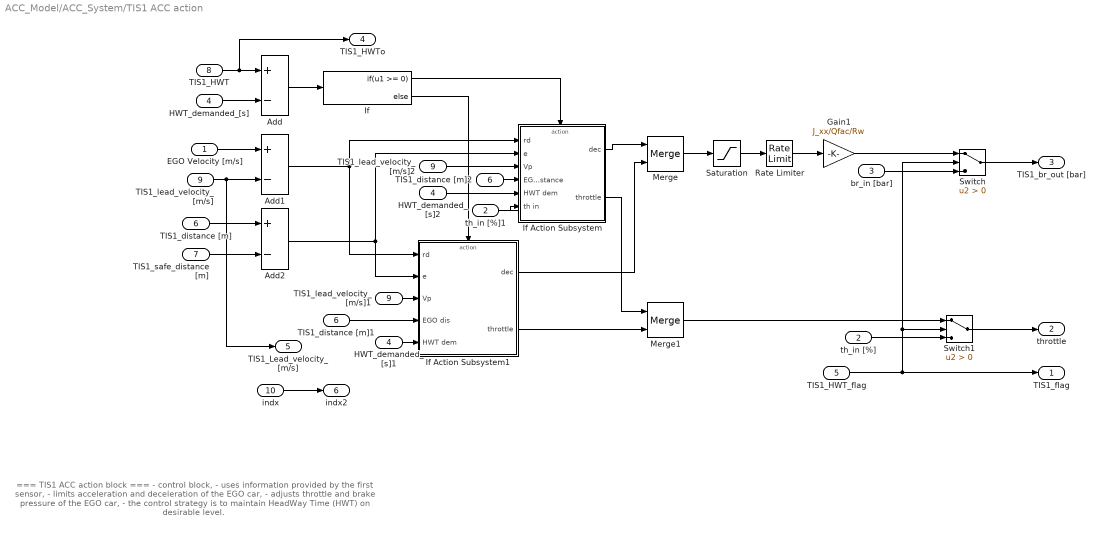
== system ACC_Model/ACC_System/TIS1 ACC action ==
  note: === TIS1 ACC action block ===
      |
      |  - control block,
      |  - uses information provided by the first sensor,
      |  - limits acceleration and deceleration of the EGO car,
      |  - adjusts throttle and brake pressure of the EGO car,
      |  - the control strategy is to maintain HeadWay Time (HWT)
      |    on desirable level.
  EGO Velocity [m/s] : Inport
  th_in [%] : Inport  Port=2
  br_in [bar] : Inport  Port=3
  HWT_demanded_[s] : Inport  Port=4
  TIS1_HWT_flag : Inport  Port=5
  TIS1_distance [m] : Inport  Port=6
  TIS1_safe_distance [m] : Inport  Port=7
  TIS1_HWT : Inport  Port=8
  TIS1_lead_velocity_[m/s] : Inport  Port=9
  indx : Inport  Port=10
  Add : Sum  Inputs=+-
  Add1 : Sum  Inputs=+-
  Add2 : Sum  Inputs=+-
  Gain1 : Gain  Gain=J_xx/Qfac/Rw
  HWT_demanded_[s]1 : InportShadow  Port=4
  HWT_demanded_[s]2 : InportShadow  Port=4
  If : If  IfExpression=u1 >= 0  SampleTime=Tsensor
  If Action Subsystem : Subsystem  TreatAsAtomicUnit=on
  If Action Subsystem1 : Subsystem  TreatAsAtomicUnit=on
  Merge : Merge
  Merge1 : Merge
  Rate Limiter : RateLimiter  RisingSlewLimit=BrakeMax  FallingSlewLimit=-BrakeMax  SampleTimeMode=inherited
  Saturation : Saturate  UpperLimit=BrakeMax  LowerLimit=0
  Switch : Switch  Criteria=u2 > Threshold
  Switch1 : Switch  Criteria=u2 > Threshold
  TIS1_distance [m]1 : InportShadow  Port=6
  TIS1_distance [m]2 : InportShadow  Port=6
  TIS1_lead_velocity_[m/s]1 : InportShadow  Port=9
  TIS1_lead_velocity_[m/s]2 : InportShadow  Port=9
  th_in [%]1 : InportShadow  Port=2
  TIS1_flag : Outport
  throttle : Outport  Port=2
  TIS1_br_out [bar] : Outport  Port=3
  TIS1_HWTo : Outport  Port=4
  TIS1_Lead_velocity_[m/s] : Outport  Port=5
  indx2 : Outport  Port=6
  wires:
  TIS1_HWT/1 -> Add/1, TIS1_HWTo/1
  HWT_demanded_[s]/1 -> Add/2
  Add/1 -> If/1
  If/1 -> If Action Subsystem/Action
  If/2 -> If Action Subsystem1/Action
  EGO Velocity [m/s]/1 -> Add1/1
  TIS1_lead_velocity_[m/s]/1 -> Add1/2, TIS1_Lead_velocity_[m/s]/1
  Add1/1 -> If Action Subsystem/1(rd), If Action Subsystem1/1(rd)
  TIS1_distance [m]/1 -> Add2/1
  TIS1_safe_distance [m]/1 -> Add2/2
  Add2/1 -> If Action Subsystem1/2(e), If Action Subsystem/2(e)
  If Action Subsystem/1(dec) -> Merge/1
  If Action Subsystem1/1(dec) -> Merge/2
  If Action Subsystem/2(throttle) -> Merge1/1
  If Action Subsystem1/2(throttle) -> Merge1/2
  Saturation/1 -> Rate Limiter/1
  Merge/1 -> Saturation/1
  TIS1_HWT_flag/1 -> TIS1_flag/1, Switch1/2, Switch/2
  Switch/1 -> TIS1_br_out [bar]/1
  Switch1/1 -> throttle/1
  Gain1/1 -> Switch/1
  Merge1/1 -> Switch1/1
  br_in [bar]/1 -> Switch/3
  th_in [%]/1 -> Switch1/3
  TIS1_distance [m]1/1 -> If Action Subsystem1/4(EGO dis)
  TIS1_lead_velocity_[m/s]1/1 -> If Action Subsystem1/3(Vp)
  HWT_demanded_[s]1/1 -> If Action Subsystem1/5(HWT dem)
  TIS1_lead_velocity_[m/s]2/1 -> If Action Subsystem/3(Vp)
  TIS1_distance [m]2/1 -> If Action Subsystem/4(EGO distance)
  HWT_demanded_[s]2/1 -> If Action Subsystem/5(HWT dem)
  th_in [%]1/1 -> If Action Subsystem/6(th in)
  indx/1 -> indx2/1
  Rate Limiter/1 -> Gain1/1

== system ACC_Model/ACC_System/TIS1 Bend Road ==
  note: === TIS1 Bend Road block ===
      |
      |  - interpretes information provided from the first TIS sensor,
      |  - computes HeadWay Time (HWT) for object on the lane of the EGO car on the bend road,
      |  - determines if detected objects is potentially dengerous,
      |  - outputs distance to the following car, computes its velocity and safe distance to be kept.
  EGO_velocity [m/s] : Inport
  TIS1_range [m] : Inport  Port=2  PortDimensions=TISdet(1)
  TIS1_rangedot [m/s] : Inport  Port=3  PortDimensions=TISdet(1)
  TIS1_theta [deg] : Inport  Port=4  PortDimensions=TISdet(1)
  HWT_dem [s] : Inport  Port=5
  Standstill [m] : Inport  Port=6
  EGO_Yaw_rate [deg/s] : Inport  Port=7
  EGO_velocity [m/s]2 : InportShadow  Port=1
  Embedded MATLAB Function : Stateflow chart  TreatAsAtomicUnit=on
  Hold : Subsystem
  Lead Car Longitudinal Velocity : Subsystem
  TIS1 Closest Object On Bend Road : Subsystem
  TIS1 HWT Computing : Subsystem
  TIS1 HWT Flag : Subsystem
  TIS1 Objects On Bend Road : Subsystem
  TIS1 Sorting  Fun : Subsystem
  HWT_flag : Outport
  TIS1 Lead distance [m] : Outport  Port=2
  TIS1 Safe_distance [m] : Outport  Port=3
  TIS1_HWT_bend : Outport  Port=4
  TIS1 lead velocity [m/s] : Outport  Port=5
  index : Outport  Port=6
  wires:
  TIS1_theta [deg]/1 -> TIS1 Sorting  Fun/3(TIS1theta [deg])
  TIS1_rangedot [m/s]/1 -> TIS1 Sorting  Fun/2(TIS1rangedot [m/s])
  TIS1_range [m]/1 -> TIS1 Sorting  Fun/1(TIS1range [m])
  TIS1 Sorting  Fun/1(TIS1_RANGE [m]) -> TIS1 Objects On Bend Road/1(TIS1_range [m])
  TIS1 Sorting  Fun/2(TIS1_RANGEDOT [m/s]) -> TIS1 Objects On Bend Road/2(TIS1_rangedot [m/s])
  TIS1 Sorting  Fun/3(TIS1_THETA [rad]) -> TIS1 Objects On Bend Road/3(TIS1_theta [rad])
  EGO_velocity [m/s]/1 -> TIS1 Objects On Bend Road/4(EGO_Velocity [m/s])
  EGO_Yaw_rate [deg/s]/1 -> TIS1 Objects On Bend Road/5(EGO_Yaw_rate_[deg/s])
  Embedded MATLAB Function/1(index) -> TIS1 Closest Object On Bend Road/1(index), index/1
  TIS1 Objects On Bend Road/1(TIS1_RANGE [m]) -> TIS1 Closest Object On Bend Road/2(TIS1_range [m]), Embedded MATLAB Function/1(distance)
  TIS1 Objects On Bend Road/2(TIS1_RANGEDOT [m/s]) -> TIS1 Closest Object On Bend Road/3(TIS1_rangedot [m])
  TIS1 Objects On Bend Road/3(TIS1_THETA [rad]) -> TIS1 Closest Object On Bend Road/4(TIS1_theta [rad])
  TIS1 Objects On Bend Road/4(TIS1_Distance [m]) -> TIS1 Closest Object On Bend Road/5(TIS1_Distance [m])
  TIS1 Objects On Bend Road/5(TIS1_lambda_[rad]) -> TIS1 Closest Object On Bend Road/6(TIS1_lambda [rad])
  TIS1 Closest Object On Bend Road/4(Distance [m]) -> TIS1 Lead distance [m]/1, TIS1 HWT Computing/1(Distance [m]), TIS1 HWT Flag/1(Distance closest [m])
  EGO_velocity [m/s]2/1 -> Lead Car Longitudinal Velocity/3(EGO Velocity [m/s]), TIS1 HWT Computing/2(Velocity [m/s])
  TIS1 Closest Object On Bend Road/2(rangedot [m/s]) -> Lead Car Longitudinal Velocity/2(TIS1 Rangedot [m/s])
  TIS1 HWT Computing/1(HWT [s]) -> TIS1_HWT_bend/1, TIS1 HWT Flag/2(HWT [s])
  HWT_dem [s]/1 -> Lead Car Longitudinal Velocity/1(HWT_dem (s)), TIS1 HWT Flag/3(HWT_dem [s])
  Standstill [m]/1 -> Lead Car Longitudinal Velocity/4(Standstill [m]), TIS1 HWT Flag/4(Standstill distance)
  TIS1 Closest Object On Bend Road/3(theta [rad]) -> Lead Car Longitudinal Velocity/5(theta [rad])
  TIS1 Closest Object On Bend Road/5(lambda [rad]) -> Lead Car Longitudinal Velocity/6(lambda [rad])
  Lead Car Longitudinal Velocity/1(Safe distance [m]) -> TIS1 Safe_distance [m]/1
  Lead Car Longitudinal Velocity/2(Lead velocity [m/s]) -> TIS1 lead velocity [m/s]/1, Hold/2(lead_vel_in)
  Hold/1(HWT_flag) -> HWT_flag/1
  TIS1 HWT Flag/1(HWT_flag) -> Hold/1(HWTflagIN)
  TIS1 Closest Object On Bend Road/1(range [m]) -> Lead Car Longitudinal Velocity/7(TIS1 Range [m])

== system ACC_Model/ACC_System/TIS1 Straight Road ==
  note: === TIS1 Straight Road block ===
      |
      |  - interpretes information provided from the first TIS sensor,
      |  - computes HeadWay Time (HWT) for object on the lane in front of the EGO car,
      |  - determines if detected objects is potentially dengerous,
      |  - outputs distance to the following car, computes its velocity and safe distance to be kept.
  EGO_velocity [m/s] : Inport
  TIS1_range [m] : Inport  Port=2  PortDimensions=TISdet(1)
  TIS1_rangedot [m/s] : Inport  Port=3  PortDimensions=TISdet(1)
  TIS1_theta [deg] : Inport  Port=4  PortDimensions=TISdet(1)
  HWT_dem [s] : Inport  Port=5
  Standstill [m] : Inport  Port=6
  HWT_dem [s]1 : InportShadow  Port=5
  Hold : Subsystem
  TIS1 Closest Object : Subsystem
  TIS1 HWT Computing : Subsystem
  TIS1 HWT Computing1 : Subsystem
  TIS1 HWT Flag : Subsystem
  TIS1 Lead Car Longitudinal Velocity : Subsystem
  TIS1 Objects On Lane : Subsystem
  TIS1 Sorting Fun : Subsystem
  TIS1_closest_object_search : Stateflow chart  TreatAsAtomicUnit=on
  HWT_flag : Outport
  TIS1 Lead distance [m] : Outport  Port=2
  TIS1 Safe_distance [m] : Outport  Port=3
  TIS1_HWT_straight : Outport  Port=4
  TIS1 Lead velocity [m/s] : Outport  Port=5
  index : Outport  Port=6
  wires:
  TIS1_range [m]/1 -> TIS1 Sorting Fun/1(TIS1range [m])
  TIS1_rangedot [m/s]/1 -> TIS1 Sorting Fun/2(TIS1rangedot [m/s])
  TIS1_theta [deg]/1 -> TIS1 Sorting Fun/3(TIS1theta [deg])
  TIS1 Sorting Fun/1(TIS1_RANGE [m]) -> TIS1 Objects On Lane/1(TIS1_range [m])
  TIS1 Sorting Fun/2(TIS1_RANGEDOT [m/s]) -> TIS1 Objects On Lane/2(TIS1_rangedot [m/s])
  TIS1 Sorting Fun/3(TIS1_THETA [rad]) -> TIS1 Objects On Lane/3(TIS1_theta [rad])
  TIS1_closest_object_search/1(index) -> TIS1 Closest Object/3(index), index/1
  TIS1 HWT Computing/1(HWT [s]) -> TIS1 HWT Flag/3(HWT [s])
  HWT_dem [s]/1 -> TIS1 Lead Car Longitudinal Velocity/1(HWT_dem (s)), TIS1 HWT Flag/2(HWT_dem [s])
  TIS1 Objects On Lane/1(TIS1_RANGEDOT [m/s]) -> TIS1 Closest Object/1(TIS1_rangedot [m/s])
  Standstill [m]/1 -> TIS1 Lead Car Longitudinal Velocity/4(Standstill [m]), TIS1 HWT Flag/4(Standstill distance)
  EGO_velocity [m/s]/1 -> TIS1 Lead Car Longitudinal Velocity/3(EGO Velocity [m/s]), TIS1 HWT Computing1/2(Velocity [m/s]), TIS1 HWT Computing/3(Velocity [m/s])
  TIS1 Closest Object/1(rangedot [m/s]) -> TIS1 Lead Car Longitudinal Velocity/2(TIS1 Rangedot [m/s])
  TIS1 Closest Object/2(Distance [m/s]) -> TIS1 Lead distance [m]/1, TIS1 HWT Computing1/1(Distance [m]), TIS1 HWT Flag/1(Distance closest [m])
  HWT_dem [s]1/1 -> TIS1 HWT Computing/2(HWT demanded)
  TIS1 HWT Computing1/1(HWT [s]) -> TIS1_HWT_straight/1
  TIS1 HWT Flag/1(HWT_flag) -> Hold/1(HWTflagIN)
  TIS1 Lead Car Longitudinal Velocity/1(lead_velocity [m/s]) -> Hold/2(lead_vel_in), TIS1 Lead velocity [m/s]/1
  TIS1 Lead Car Longitudinal Velocity/2(Safe distance [m]) -> TIS1 Safe_distance [m]/1
  Hold/1(HWT_flag) -> HWT_flag/1
  TIS1 Objects On Lane/2(TIS1_Distance [m]) -> TIS1 Closest Object/2(TIS1_Distance [m]), TIS1 HWT Computing/1(Distance [m]), TIS1_closest_object_search/1(distance)

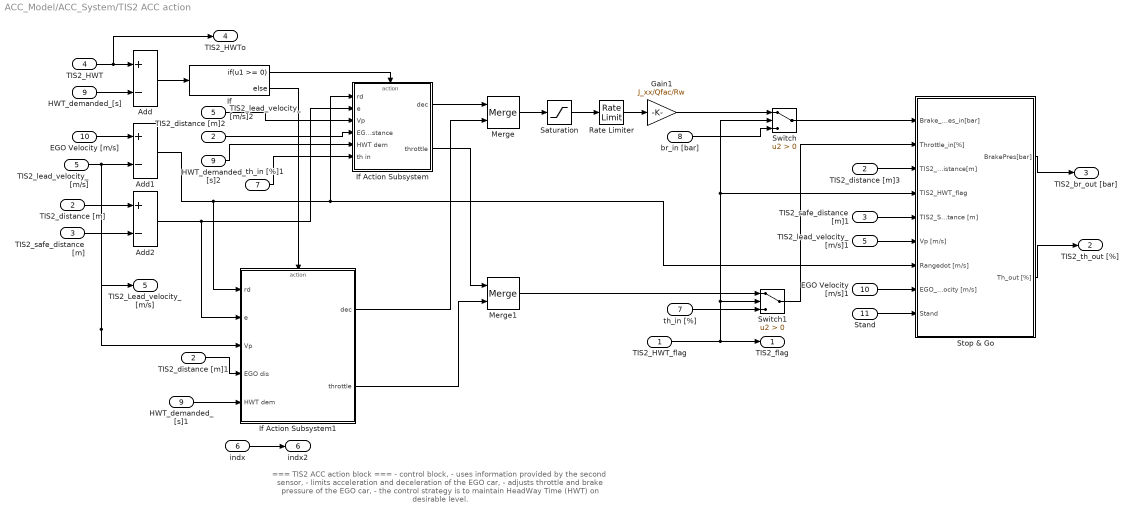
== system ACC_Model/ACC_System/TIS2 ACC action ==
  note: === TIS2 ACC action block ===
      |
      |  - control block,
      |  - uses information provided by the second sensor,
      |  - limits acceleration and deceleration of the EGO car,
      |  - adjusts throttle and brake pressure of the EGO car,
      |  - the control strategy is to maintain HeadWay Time (HWT)
      |    on desirable level.
  TIS2_HWT_flag : Inport
  TIS2_distance [m] : Inport  Port=2
  TIS2_safe_distance [m] : Inport  Port=3
  TIS2_HWT : Inport  Port=4
  TIS2_lead_velocity_[m/s] : Inport  Port=5
  indx : Inport  Port=6
  th_in [%] : Inport  Port=7
  br_in [bar] : Inport  Port=8
  HWT_demanded_[s] : Inport  Port=9
  EGO Velocity [m/s] : Inport  Port=10
  Stand : Inport  Port=11
  Add : Sum  Inputs=+-
  Add1 : Sum  Inputs=+-
  Add2 : Sum  Inputs=+-
  EGO Velocity [m/s]1 : InportShadow  Port=10
  Gain1 : Gain  Gain=J_xx/Qfac/Rw
  HWT_demanded_[s]1 : InportShadow  Port=9
  HWT_demanded_[s]2 : InportShadow  Port=9
  If : If  IfExpression=u1 >= 0
  If Action Subsystem : Subsystem  TreatAsAtomicUnit=on
  If Action Subsystem1 : Subsystem  TreatAsAtomicUnit=on
  Merge : Merge
  Merge1 : Merge
  Rate Limiter : RateLimiter  RisingSlewLimit=BrakeMax  FallingSlewLimit=-BrakeMax  SampleTimeMode=inherited
  Saturation : Saturate  UpperLimit=BrakeMax  LowerLimit=0
  Stop & Go : Subsystem
  Switch : Switch  Criteria=u2 > Threshold
  Switch1 : Switch  Criteria=u2 > Threshold
  TIS2_distance [m]1 : InportShadow  Port=2
  TIS2_distance [m]2 : InportShadow  Port=2
  TIS2_distance [m]3 : InportShadow  Port=2
  TIS2_lead_velocity_[m/s]1 : InportShadow  Port=5
  TIS2_lead_velocity_[m/s]2 : InportShadow  Port=5
  TIS2_safe_distance [m]1 : InportShadow  Port=3
  th_in [%]1 : InportShadow  Port=7
  TIS2_flag : Outport
  TIS2_th_out [%] : Outport  Port=2
  TIS2_br_out [bar] : Outport  Port=3
  TIS2_HWTo : Outport  Port=4
  TIS2_Lead_velocity_[m/s] : Outport  Port=5
  indx2 : Outport  Port=6
  wires:
  TIS2_HWT/1 -> Add/1, TIS2_HWTo/1
  HWT_demanded_[s]/1 -> Add/2
  Add/1 -> If/1
  EGO Velocity [m/s]/1 -> Add1/1
  TIS2_lead_velocity_[m/s]/1 -> Add1/2, If Action Subsystem1/3(Vp), TIS2_Lead_velocity_[m/s]/1
  Add1/1 -> If Action Subsystem/1(rd), Stop & Go/7(Rangedot [m/s]), If Action Subsystem1/1(rd)
  TIS2_distance [m]/1 -> Add2/1
  TIS2_safe_distance [m]/1 -> Add2/2
  Saturation/1 -> Rate Limiter/1
  Merge/1 -> Saturation/1
  TIS2_HWT_flag/1 -> Switch1/2, Switch/2, Stop & Go/4(TIS2_HWT_flag), TIS2_flag/1
  Switch1/1 -> Stop & Go/2(Throttle_in[%])
  Gain1/1 -> Switch/1
  Merge1/1 -> Switch1/1
  br_in [bar]/1 -> Switch/3
  th_in [%]/1 -> Switch1/3
  Switch/1 -> Stop & Go/1(Brake_Pres_in[bar])
  TIS2_distance [m]3/1 -> Stop & Go/3(TIS2_Distance[m])
  Stop & Go/2(Th_out [%]) -> TIS2_th_out [%]/1
  Stop & Go/1(BrakePres[bar]) -> TIS2_br_out [bar]/1
  TIS2_safe_distance [m]1/1 -> Stop & Go/5(TIS2_Safe_Distance [m])
  EGO Velocity [m/s]1/1 -> Stop & Go/8(EGO_Velocity [m/s])
  If/1 -> If Action Subsystem/Action
  If/2 -> If Action Subsystem1/Action
  If Action Subsystem/1(dec) -> Merge/1
  If Action Subsystem1/1(dec) -> Merge/2
  If Action Subsystem/2(throttle) -> Merge1/1
  If Action Subsystem1/2(throttle) -> Merge1/2
  Add2/1 -> If Action Subsystem1/2(e), If Action Subsystem/2(e)
  th_in [%]1/1 -> If Action Subsystem/6(th in)
  Stand/1 -> Stop & Go/9(Stand)
  HWT_demanded_[s]1/1 -> If Action Subsystem1/5(HWT dem)
  TIS2_distance [m]1/1 -> If Action Subsystem1/4(EGO dis)
  TIS2_lead_velocity_[m/s]1/1 -> Stop & Go/6(Vp [m/s])
  HWT_demanded_[s]2/1 -> If Action Subsystem/5(HWT dem)
  TIS2_distance [m]2/1 -> If Action Subsystem/4(EGO distance)
  TIS2_lead_velocity_[m/s]2/1 -> If Action Subsystem/3(Vp)
  indx/1 -> indx2/1
  Rate Limiter/1 -> Gain1/1

== system ACC_Model/ACC_System/TIS2 Bend Road ==
  note: === TIS2 Bend Road block ===
      |
      |  - interpretes information provided from the first TIS sensor,
      |  - computes HeadWay Time (HWT) for object on the lane of the EGO car on the bend road,
      |  - determines if detected objects is potentially dengerous,
      |  - outputs distance to the following car, computes its velocity and safe distance to be kept.
  EGO_velocity [m/s] : Inport
  TIS2_range [m] : Inport  Port=2  PortDimensions=TISdet(2)
  TIS2_rangedot [m/s] : Inport  Port=3  PortDimensions=TISdet(2)
  TIS2_theta [deg] : Inport  Port=4  PortDimensions=TISdet(2)
  HWT_dem [s] : Inport  Port=5
  Standstill [m] : Inport  Port=6
  EGO_Yaw_rate [deg/s] : Inport  Port=7
  EGO_velocity [m/s]2 : InportShadow  Port=1
  Hold : Subsystem
  Lead Car Longitudinal Velocity : Subsystem
  TIS1 HWT Computing : Subsystem
  TIS2 Closest Object On Bend Road : Subsystem
  TIS2 HWT Flag : Subsystem
  TIS2 Objects On Bend Road : Subsystem
  TIS2 Sorting Fun : Subsystem
  TIS2_closest_object_search1 : Stateflow chart  TreatAsAtomicUnit=on
  HWT_flag : Outport
  TIS2 Lead distance [m] : Outport  Port=2
  TIS2 Safe_distance [m] : Outport  Port=3
  TIS2_HWT_bend : Outport  Port=4
  TIS2 Lead velocity [m/s] : Outport  Port=5
  index : Outport  Port=6
  wires:
  TIS2_range [m]/1 -> TIS2 Sorting Fun/1(TIS2range [m])
  TIS2_rangedot [m/s]/1 -> TIS2 Sorting Fun/2(TIS2rangedot [m/s])
  TIS2_theta [deg]/1 -> TIS2 Sorting Fun/3(TIS2theta [deg])
  TIS2 Sorting Fun/1(TIS2_RANGE [m]) -> TIS2 Objects On Bend Road/1(TIS2_range [m])
  TIS2 Sorting Fun/2(TIS2_RANGEDOT [m/s]) -> TIS2 Objects On Bend Road/2(TIS2_rangedot [m/s])
  TIS2 Sorting Fun/3(TIS2_THETA [rad]) -> TIS2 Objects On Bend Road/3(TIS2_theta [rad])
  TIS2 Objects On Bend Road/1(TIS2_RANGE [m]) -> TIS2 Closest Object On Bend Road/2(TIS2_range [m]), TIS2_closest_object_search1/1(distance)
  TIS2 Objects On Bend Road/2(TIS2_RANGEDOT [m/s]) -> TIS2 Closest Object On Bend Road/3(TIS2_rangedot [m])
  TIS2 Objects On Bend Road/3(TIS2_THETA [rad]) -> TIS2 Closest Object On Bend Road/4(TIS2_theta [rad])
  TIS2 Objects On Bend Road/4(TIS1_Distance [m]) -> TIS2 Closest Object On Bend Road/5(TIS2_Distance [m])
  TIS2 Objects On Bend Road/5(TIS2_lambda_[rad]) -> TIS2 Closest Object On Bend Road/6(TIS2_lambda [rad])
  EGO_Yaw_rate [deg/s]/1 -> TIS2 Objects On Bend Road/5(EGO_Yaw_rate_[deg/s])
  EGO_velocity [m/s]/1 -> TIS2 Objects On Bend Road/4(EGO_Velocity [m/s])
  TIS2_closest_object_search1/1(index) -> TIS2 Closest Object On Bend Road/1(index), index/1
  TIS2 Closest Object On Bend Road/3(Distance [m]) -> TIS2 Lead distance [m]/1, TIS2 HWT Flag/1(Distance closest [m]), TIS1 HWT Computing/1(Distance [m])
  EGO_velocity [m/s]2/1 -> TIS1 HWT Computing/2(Velocity [m/s]), Lead Car Longitudinal Velocity/3(EGO Velocity [m/s])
  TIS2 Closest Object On Bend Road/1(rangedot [m/s]) -> Lead Car Longitudinal Velocity/2(TIS1 Rangedot [m/s])
  HWT_dem [s]/1 -> Lead Car Longitudinal Velocity/1(HWT_dem (s)), TIS2 HWT Flag/3(HWT_dem [s])
  TIS1 HWT Computing/1(HWT [s]) -> TIS2_HWT_bend/1, TIS2 HWT Flag/2(HWT [s])
  Standstill [m]/1 -> Lead Car Longitudinal Velocity/4(Standstill [m]), TIS2 HWT Flag/4(Standstill distance)
  TIS2 Closest Object On Bend Road/5(lambda [rad]) -> Lead Car Longitudinal Velocity/6(lambda [rad])
  TIS2 Closest Object On Bend Road/2(theta [rad]) -> Lead Car Longitudinal Velocity/5(theta [rad])
  TIS2 Closest Object On Bend Road/4(range [m]) -> Lead Car Longitudinal Velocity/7(TIS2 Range [m])
  Lead Car Longitudinal Velocity/1(Safe distance [m]) -> TIS2 Safe_distance [m]/1
  Lead Car Longitudinal Velocity/2(Lead velocity [m/s]) -> TIS2 Lead velocity [m/s]/1, Hold/2(lead_vel_in)
  Hold/1(HWT_flag) -> HWT_flag/1
  TIS2 HWT Flag/1(HWT_flag) -> Hold/1(HWTflagIN)
